simulink model "BoxcarAveragerFixedPoint"  (R2023b)
settings: Solver=FixedStepDiscrete  StartTime=0.0  StopTime=0.001  RelTol=1e-3
model workspace (MAT data in the model file):
  test = 0
undefined symbols (not defined in the file): a, b, c
libraries: hdlsllib x4, dspsrcs4 x1
settings Model: DataTypeOverride=Off  FPTShortcutValueString='{{},{''BaselineRun'',1,1,1,''BaselineRun'','''',{},''M'',''F'',''''},{''EmbeddedRun'',1,1,1,''EmbeddedRun'','''',{},''M'','''',''''},{''BaselineRun_5'',1,1,1,''BaselineRun_5'','''',{},''M'',''F'',''''}}'  Creator=max_d  LastModifiedBy=heyan
settings SolverCC: AlgebraicLoopSolver=TrustRegion  AutoInsertRateTranBlk=on
settings DataIOCC: LimitDataPoints=on  SaveOutput=off  SaveTime=off
settings OptimizationCC: BlockReduction=off  ConditionallyExecuteInputs=off  DefaultParameterBehavior=Inlined  InheritOutputTypeSmallerThanSingle=on  LifeSpan=inf
settings DebuggingCC: SignalRangeChecking=warning  AlgebraicLoopMsg=error  SingleTaskRateTransMsg=error  UnconnectedInputMsg=warning  UnconnectedOutputMsg=warning  UnconnectedLineMsg=warning  AllowSymbolicDim=off  StrictBusMsg=ErrorOnBusTreatedAsVector  SFUnexpectedBacktrackingDiag=warning  SFNoUnconditionalDefaultTransitionDiag=warning  SFExecutionAtInitializationDiag=none  ArithmeticOperatorsInVariantConditions=warning
settings HardwareCC: ProdBitPerPointer=32  ProdBitPerSizeT=32  ProdBitPerPtrDiffT=32  ProdLargestAtomicFloat=None  ProdIntDivRoundTo=Undefined  ProdEndianess=Unspecified  ProdWordSize=32  ProdHWDeviceType=ASIC/FPGA->ASIC/FPGA  ProdEqTarget=off
settings ModelReferenceCC: EnableRefExpFcnMdlSchedulingChecks=on
settings SFSimCC: SimUseLocalCustomCode=off  CustomCodeUndefinedFunction=UseInterfaceOnly
settings RTWCC: RTWUseLocalCustomCode=off  DLArmComputeVersion=19.05
settings CodeAppCC: StateflowObjectComments=on
settings GRTTargetCC: TargetLangStandard=C89/C90 (ANSI)
settings ConfigComp: CovScope=ReferencedModels  CovMetricSettings=dw  CovSaveCumulativeToWorkspaceVar=on  CovSaveSingleToWorkspaceVar=on  CovExternalEMLEnable=off  CovSFcnEnable=off

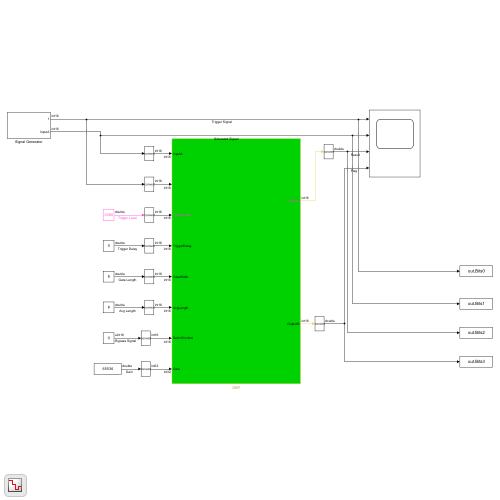
[thumbnail: Simulink's stored preview of the top-level diagram]
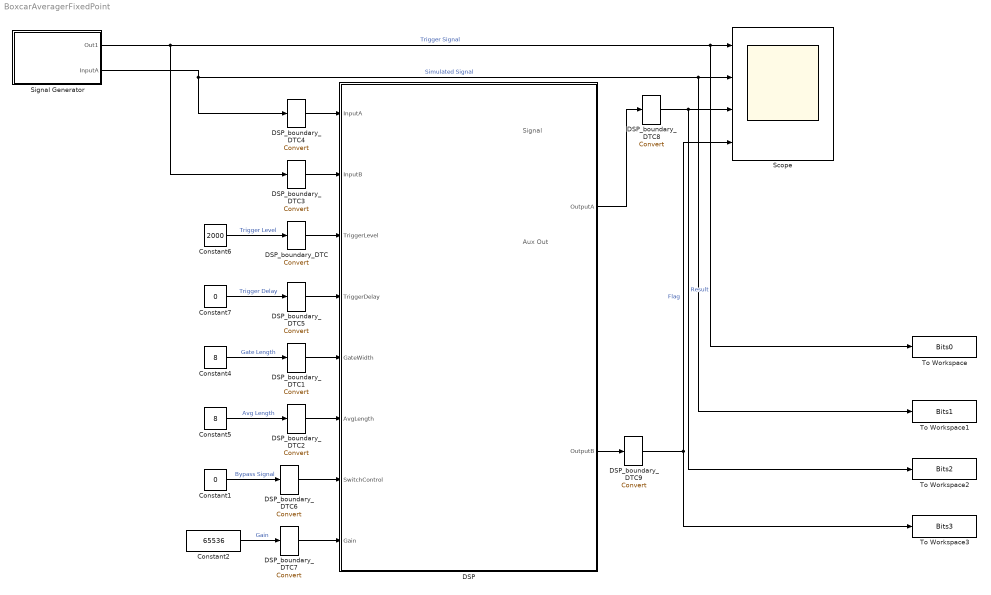
== system BoxcarAveragerFixedPoint ==
  note: Signal
  note: Aux Out
  Constant1 : Constant  Value=0  OutDataTypeStr=fixdt(0,16,0)  SampleTime=1/312.5e6
  Constant2 : Constant  Value=65536  OutDataTypeStr=double  SampleTime=1/312.5e6
  Constant4 : Constant  Value=8  OutDataTypeStr=double  SampleTime=1/312.5e6
  Constant5 : Constant  Value=8  OutDataTypeStr=double  SampleTime=1/312.5e6
  Constant6 : Constant  Value=2000  OutDataTypeStr=double  SampleTime=1/312.5e6
  Constant7 : Constant  Value=0  OutDataTypeStr=double  SampleTime=1/312.5e6
  DSP : Subsystem
  DSP_boundary_DTC{,1..9} (10 alike) : DataTypeConversion
  Scope : Scope  NumInputPorts=4
  Signal Generator : Subsystem
  To Workspace : ToWorkspace  VariableName=Bits0  SampleTime=-1
      settings: Save2DSignal=2-D array (concatenate along first dimension)
  To Workspace1 : ToWorkspace  VariableName=Bits1  SampleTime=-1
      settings: Save2DSignal=2-D array (concatenate along first dimension)
  To Workspace2 : ToWorkspace  VariableName=Bits2  SampleTime=-1
      settings: Save2DSignal=2-D array (concatenate along first dimension)
  To Workspace3 : ToWorkspace  VariableName=Bits3  SampleTime=-1
      settings: Save2DSignal=2-D array (concatenate along first dimension)
  wires:
  Constant2/1 -> DSP_boundary_DTC7/1  "Gain"
  Constant1/1 -> DSP_boundary_DTC6/1  "Bypass Signal"
  Constant5/1 -> DSP_boundary_DTC2/1  "Avg Length"
  Constant4/1 -> DSP_boundary_DTC1/1  "Gate Length"
  Constant7/1 -> DSP_boundary_DTC5/1  "Trigger Delay"
  Constant6/1 -> DSP_boundary_DTC/1  "Trigger Level"
  Signal Generator/1(Out1) -> DSP_boundary_DTC3/1, To Workspace/1, Scope/1  "Trigger Signal"
  Signal Generator/2(InputA) -> DSP_boundary_DTC4/1, To Workspace1/1, Scope/2  "Simulated Signal"
  DSP/1(OutputA) -> DSP_boundary_DTC8/1
  DSP/2(OutputB) -> DSP_boundary_DTC9/1
  DSP_boundary_DTC/1 -> DSP/3(TriggerLevel)
  DSP_boundary_DTC1/1 -> DSP/5(GateWidth)
  DSP_boundary_DTC2/1 -> DSP/6(AvgLength)
  DSP_boundary_DTC3/1 -> DSP/2(InputB)
  DSP_boundary_DTC4/1 -> DSP/1(InputA)
  DSP_boundary_DTC5/1 -> DSP/4(TriggerDelay)
  DSP_boundary_DTC7/1 -> DSP/8(Gain)
  DSP_boundary_DTC6/1 -> DSP/7(SwitchControl)
  DSP_boundary_DTC8/1 -> To Workspace2/1, Scope/3  "Result"
  DSP_boundary_DTC9/1 -> Scope/4, To Workspace3/1  "Flag"

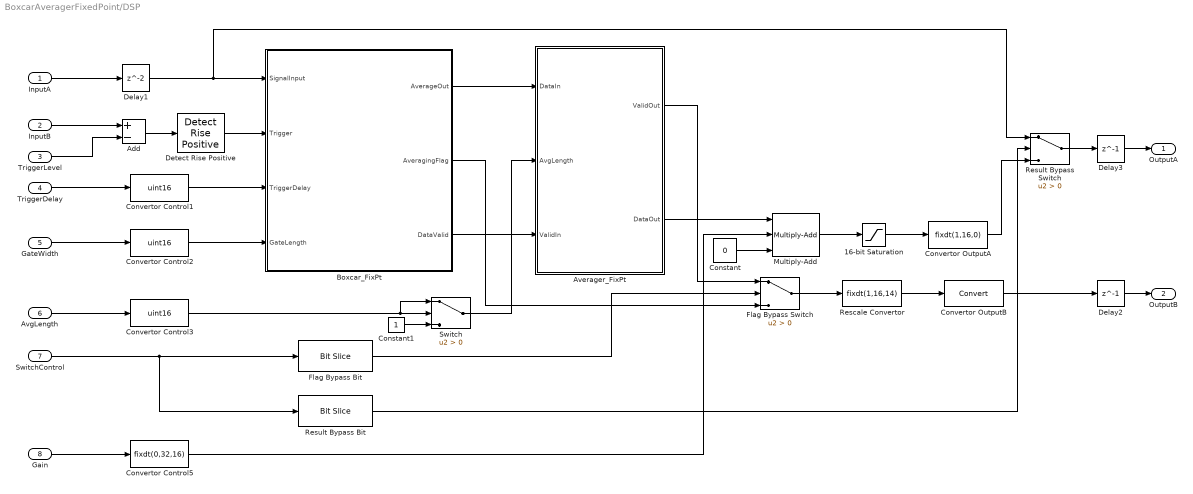
== system BoxcarAveragerFixedPoint/DSP ==
  InputA : Inport  OutDataTypeStr=fixdt(1,16,0)
  InputB : Inport  Port=2  OutDataTypeStr=fixdt(1,16,0)
  TriggerLevel : Inport  Port=3  OutDataTypeStr=fixdt(1,16,0)
  TriggerDelay : Inport  Port=4  OutDataTypeStr=fixdt(1,16,0)
  GateWidth : Inport  Port=5  OutDataTypeStr=fixdt(1,16,0)
  AvgLength : Inport  Port=6  OutDataTypeStr=fixdt(1,16,0)
  SwitchControl : Inport  Port=7  OutDataTypeStr=fixdt(1,16,0)
  Gain : Inport  Port=8  OutDataTypeStr=fixdt(1,32,0)
  16-bit Saturation : Saturate  UpperLimit=32767  LowerLimit=-32768  OutDataTypeStr=fixdt(1,81,16)
  Add : Sum  Inputs=+-  OutDataTypeStr=fixdt(1,17,0)
  Averager_FixPt : MATLAB Function  TreatAsAtomicUnit=on  VariantControl=(default)
  Boxcar_FixPt : MATLAB Function  TreatAsAtomicUnit=on  VariantControl=(default)
  Constant : Constant  Value=0  OutDataTypeStr=fixdt(0,1,0)  SampleTime=1/312.5e6
  Constant1 : Constant  OutDataTypeStr=uint16  SampleTime=-1
  Convertor Control1 : DataTypeConversion  OutDataTypeStr=uint16  ConvertRealWorld=Stored Integer (SI)  SaturateOnIntegerOverflow=off  RndMeth=Floor
  Convertor Control2 : DataTypeConversion  OutDataTypeStr=uint16  ConvertRealWorld=Stored Integer (SI)  SaturateOnIntegerOverflow=off  RndMeth=Floor
  Convertor Control3 : DataTypeConversion  OutDataTypeStr=uint16  ConvertRealWorld=Stored Integer (SI)  SaturateOnIntegerOverflow=off  RndMeth=Floor
  Convertor Control5 : DataTypeConversion  OutDataTypeStr=fixdt(0,32,16)  ConvertRealWorld=Stored Integer (SI)  SaturateOnIntegerOverflow=off  RndMeth=Floor
  Convertor OutputA : DataTypeConversion  OutDataTypeStr=fixdt(1,16,0)  SaturateOnIntegerOverflow=off  RndMeth=Floor
  Convertor OutputB : DataTypeConversion  ConvertRealWorld=Stored Integer (SI)  SaturateOnIntegerOverflow=off  RndMeth=Floor
  Delay1 : Delay  InitialCondition=0
  Delay2 : Delay  DelayLength=1  InitialCondition=0
  Delay3 : Delay  DelayLength=1  InitialCondition=0
  Detect Rise Positive : hdlsllib/Logic and Bit Operations/Detect Rise Positive  vinit=0  OutDataTypeStr=boolean
  Flag Bypass Bit : hdlsllib/Logic and Bit Operations/Bit Slice  lidx=0  ridx=0
  Flag Bypass Switch : Switch  Criteria=u2 > Threshold  OutDataTypeStr=fixdt(0,1,0)  SaturateOnIntegerOverflow=off  InputSameDT=off
  Multiply-Add : hdlsllib/HDL Operations/Multiply-Add  Function=c+(a.*b)  datatype=fixdt(1,81,16)  DoSatur=on  FMA=off
  Rescale Convertor : DataTypeConversion  OutDataTypeStr=fixdt(1,16,14)  SaturateOnIntegerOverflow=off  RndMeth=Floor
  Result Bypass Bit : hdlsllib/Logic and Bit Operations/Bit Slice  lidx=1  ridx=1
  Result Bypass Switch : Switch  Criteria=u2 > Threshold  OutDataTypeStr=fixdt(1,16,0)  SaturateOnIntegerOverflow=off  InputSameDT=off
  Switch : Switch  Criteria=u2 > Threshold  SaturateOnIntegerOverflow=off  InputSameDT=off  OutDataTypeStr=Inherit: Same as first input
  OutputA : Outport  OutDataTypeStr=fixdt(1,16,0)  VectorParamsAs1DForOutWhenUnconnected=off
  OutputB : Outport  Port=2  OutDataTypeStr=fixdt(1,16,0)  VectorParamsAs1DForOutWhenUnconnected=off
  wires:
  GateWidth/1 -> Convertor Control2/1
  Convertor OutputA/1 -> Result Bypass Switch/3
  Multiply-Add/1 -> 16-bit Saturation/1
  Constant/1 -> Multiply-Add/3
  Rescale Convertor/1 -> Convertor OutputB/1
  TriggerLevel/1 -> Add/2
  Convertor Control2/1 -> Boxcar_FixPt/4(GateLength)
  Convertor Control3/1 -> Switch/1, Switch/2
  Add/1 -> Detect Rise Positive/1
  16-bit Saturation/1 -> Convertor OutputA/1
  Gain/1 -> Convertor Control5/1
  Averager_FixPt/2(DataOut) -> Multiply-Add/1
  Result Bypass Bit/1 -> Result Bypass Switch/2
  Flag Bypass Switch/1 -> Rescale Convertor/1
  Detect Rise Positive/1 -> Boxcar_FixPt/2(Trigger)
  Boxcar_FixPt/1(AverageOut) -> Averager_FixPt/1(DataIn)
  Convertor Control5/1 -> Multiply-Add/2
  InputA/1 -> Delay1/1
  AvgLength/1 -> Convertor Control3/1
  Convertor Control1/1 -> Boxcar_FixPt/3(TriggerDelay)
  Boxcar_FixPt/3(DataValid) -> Averager_FixPt/3(ValidIn)
  TriggerDelay/1 -> Convertor Control1/1
  InputB/1 -> Add/1
  SwitchControl/1 -> Result Bypass Bit/1, Flag Bypass Bit/1
  Delay1/1 -> Boxcar_FixPt/1(SignalInput), Result Bypass Switch/1
  Averager_FixPt/1(ValidOut) -> Flag Bypass Switch/1
  Boxcar_FixPt/2(AveragingFlag) -> Flag Bypass Switch/3
  Flag Bypass Bit/1 -> Flag Bypass Switch/2
  Constant1/1 -> Switch/3
  Switch/1 -> Averager_FixPt/2(AvgLength)
  Result Bypass Switch/1 -> Delay3/1
  Convertor OutputB/1 -> Delay2/1
  Delay2/1 -> OutputB/1
  Delay3/1 -> OutputA/1

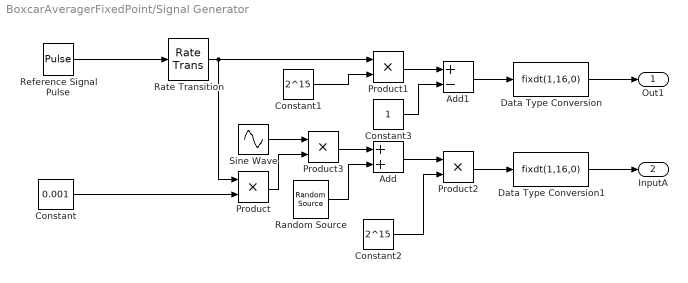
== system BoxcarAveragerFixedPoint/Signal Generator ==
  Add : Sum
  Add1 : Sum  Inputs=+-
  Constant : Constant  Value=0.001
  Constant1 : Constant  Value=2^15
  Constant2 : Constant  Value=2^15
  Constant3 : Constant
  Data Type Conversion : DataTypeConversion  OutDataTypeStr=fixdt(1,16,0)  SaturateOnIntegerOverflow=off  RndMeth=Floor
  Data Type Conversion1 : DataTypeConversion  OutDataTypeStr=fixdt(1,16,0)  SaturateOnIntegerOverflow=off  RndMeth=Floor
  Product{,1..3} (4 alike) : Product
  Random Source : dspsrcs4/Random Source  SrcType=Uniform  NormMethod=Ziggurat  CltLength=12  MinVal=-0.001  MaxVal=0.001  MeanVal=0  VarVal=1  RepMode=Not repeatable  rawSeed=1  IsInherit=off  SampMode=Discrete  SampTime=1/312.5e6  SampFrame=1  DataType=Double  OutComplex=Real  OutputFrames=off
  Rate Transition : RateTransition  OutPortSampleTime=1/312.5e6
  Reference Signal Pulse : DiscretePulseGenerator  PulseType=Time based  Period=100/(312.5e6)  PulseWidth=16
  Sine Wave : Sin  Amplitude=0.5  Bias=0.5  Frequency=2*pi*10e3  SampleTime=1/312.5e6
  Out1 : Outport  OutDataTypeStr=int16
  InputA : Outport  Port=2  OutDataTypeStr=int16
  wires:
  Data Type Conversion/1 -> Out1/1
  Reference Signal Pulse/1 -> Rate Transition/1
  Constant3/1 -> Add1/2
  Add1/1 -> Data Type Conversion/1
  Product1/1 -> Add1/1
  Product3/1 -> Add/1
  Random Source/1 -> Add/2
  Add/1 -> Product2/1
  Sine Wave/1 -> Product3/1
  Product2/1 -> Data Type Conversion1/1
  Constant2/1 -> Product2/2
  Constant/1 -> Product/2
  Product/1 -> Product3/2
  Constant1/1 -> Product1/2
  Data Type Conversion1/1 -> InputA/1
  Rate Transition/1 -> Product/1, Product1/1

== matlab function BoxcarAveragerFixedPoint/DSP/Averager_FixPt ==
  settings: fimath=fimath('RoundingMethod', 'Floor', 'OverflowAction', 'Wrap', 'ProductMode', 'FullPrecision', 'MaxProductWordLength', 128, 'SumMode', 'FullPrecision', 'MaxSumWordLength', 128)
  data: DataIn input; AvgLength input; ValidIn input; ValidOut output; DataOut output
%auto-generated
function [ValidOut,DataOut] = Average_fixpt(DataIn,AvgLength,ValidIn)
%#codegen

fm = get_fimath();
AvgLength = fi(AvgLength, 0, 16, 0, fm);
DataIn = fi(DataIn, 1, 32, 0, fm);
ValidIn = fi(ValidIn, 0, 1, 0, fm);

persistent AvgOut;
if isempty(AvgOut)
    AvgOut = fi(0, 1, 48, 0, fm);
end

persistent DataOutReg;
if isempty(DataOutReg)
    DataOutReg = fi(0, 1, 48, 0, fm);
end

persistent ValidOutReg;
if isempty(ValidOutReg)
    ValidOutReg = fi(0, 0, 1, 0, fm);
end

persistent cnt1;
if isempty(cnt1)
    cnt1 = fi(0, 0, 16, 0, fm);
end


S1 = fi(0, 0, 1, 0, fm); %Waiting for trigger
S2 = fi(1, 0, 1, 0, fm);

persistent current_state;
if isempty(current_state)
    current_state = fi(S1, 0, 1, 0, fm);   
end

switch(current_state)

    case S1
        ValidOutReg(:) = 0;
        if ValidIn == fi(1, 0, 1, 0, fm)
            current_state(:) = S2;
            cnt1(:) = fi_signed(AvgLength)-fi(1, 0, 1, 0, fm);
            AvgOut(:) = DataIn;
        else
            current_state(:) = S1;
        end

    case S2

        if ValidIn == fi(1, 0, 1, 0, fm)
            AvgOut(:) = AvgOut+DataIn;
            cnt1(:) = fi_signed(cnt1)-fi(1, 0, 1, 0, fm);
        end
        if cnt1 == fi(0, 0, 1, 0, fm)
            DataOutReg(:) = AvgOut;
            ValidOutReg(:) = 1;
            current_state(:) = S1;
        end

end

DataOut = fi(DataOutReg, 1, 48, 0, fm);
ValidOut = fi(ValidOutReg, 0, 1, 0, fm);

end



function y = fi_signed(a)
    coder.inline( 'always' );
    if isfi( a ) && ~(issigned( a ))
        nt = numerictype( a );
        new_nt = numerictype( 1, nt.WordLength + 1, nt.FractionLength );
        y = fi( a, new_nt, fimath( a ) );
    else
        y = a;
    end
end

function fm = get_fimath()
	fm = fimath('RoundingMethod', 'Floor',...
	     'OverflowAction', 'Wrap',...
	     'ProductMode','FullPrecision',...
	     'MaxProductWordLength', 128,...
	     'SumMode','FullPrecision',...
	     'MaxSumWordLength', 128);
end

== matlab function BoxcarAveragerFixedPoint/DSP/Boxcar_FixPt ==
  settings: fimath=fimath('RoundingMethod', 'Floor', 'OverflowAction', 'Wrap', 'ProductMode', 'FullPrecision', 'MaxProductWordLength', 128, 'SumMode', 'FullPrecision', 'MaxSumWordLength', 128)
  data: SignalInput input; AverageOut output; Trigger input; TriggerDelay input; GateLength input; AveragingFlag output; DataValid output
%auto-generated
%#codegen
function [AverageOut,AveragingFlag,DataValid] = Boxcar_fixpt(SignalInput, Trigger, TriggerDelay, GateLength)

fm = get_fimath();
GateLength = fi(GateLength, 0, 16, 0, fm);
SignalInput = fi(SignalInput, 1, 16, 0, fm);
TriggerDelay = fi(TriggerDelay, 0, 16, 0, fm);

persistent AvgOut;
if isempty(AvgOut)
    AvgOut = fi(0, 1, 32, 0, fm);
end


persistent cnt1;
if isempty(cnt1)
    cnt1 = fi(0, 0, 16, 0, fm);
end

persistent cnt2;
if isempty(cnt2)
    cnt2 = fi(0, 0, 16, 0, fm);
end


persistent AvgFlag;
if isempty(AvgFlag)
    AvgFlag = fi(0, 0, 1, 0, fm);
end

persistent DValid;
if isempty(DValid)
    DValid = fi(0, 0, 1, 0, fm);
end

S1 = fi(0, 0, 2, 0, fm); %Waiting for trigger
S2 = fi(1, 0, 2, 0, fm);
S3 = fi(2, 0, 2, 0, fm);

persistent current_state;
if isempty(current_state)
    current_state = fi(S1, 0, 2, 0, fm);   
end

switch(current_state)

    case S1
        DValid(:) = 0;
        AvgFlag(:) = 0;
        if Trigger == 1
            current_state(:) = S2;
            cnt1(:) = TriggerDelay;
        else
            current_state(:) = S1;
        end

    case S2

        if cnt1 == fi(0, 0, 1, 0, fm)
            current_state(:) = S3;
            cnt2(:) = GateLength;
            AvgOut(:) = 0;
        else
            cnt1(:) = fi_signed(cnt1)-fi(1, 0, 1, 0, fm);
        end

    case S3
        if cnt2 == fi(0, 0, 1, 0, fm)
            current_state(:) = S1;
            DValid(:) = 0;
        else
            AvgOut(:) = AvgOut + SignalInput;
            AvgFlag(:) = 1;
            cnt2(:) = fi_signed(cnt2)-fi(1, 0, 1, 0, fm);
            if cnt2 == fi(0, 0, 1, 0, fm)
                DValid(:) = 1;
                current_state(:) = S1;
            end 
        end

end

AverageOut = fi(AvgOut, 1, 32, 0, fm);
DataValid = fi(DValid, 0, 1, 0, fm);
AveragingFlag = fi(AvgFlag, 0, 1, 0, fm);



end



function y = fi_signed(a)
    coder.inline( 'always' );
    if isfi( a ) && ~(issigned( a ))
        nt = numerictype( a );
        new_nt = numerictype( 1, nt.WordLength + 1, nt.FractionLength );
        y = fi( a, new_nt, fimath( a ) );
    else
        y = a;
    end
end

function fm = get_fimath()
	fm = fimath('RoundingMethod', 'Floor',...
	     'OverflowAction', 'Wrap',...
	     'ProductMode','FullPrecision',...
	     'MaxProductWordLength', 128,...
	     'SumMode','FullPrecision',...
	     'MaxSumWordLength', 128);
end
